simulink model "gear_motor"  (R2015a)
settings: Solver=ode45  StartTime=0.0  StopTime=180  FixedStep=0.01  RelTol=1e-3
libraries: dsparch4 x1
settings Model: Creator=keysie  LastModifiedBy=keysie
settings GRTTargetCC: RTWCAPISignals=on  RTWCAPIParams=on

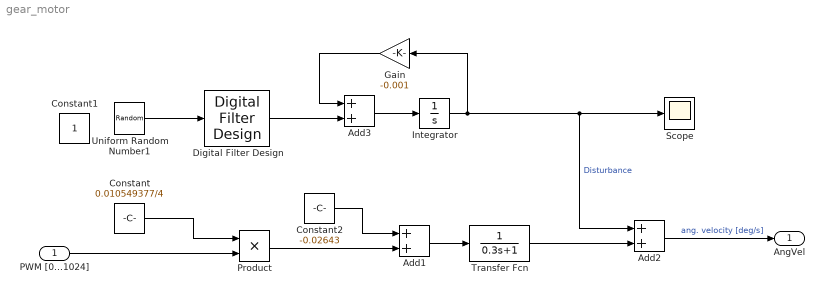
== system gear_motor ==
  PWM [0...1024] : Inport  Interpolate=off
  Add1 : Sum
  Add2 : Sum
  Add3 : Sum
  Constant : Constant  Value=0.010549377/4
  Constant2 : Constant  Value=-0.02643
  Digital Filter Design : dsparch4/Digital Filter Design  mwdsp_browser_bugfix_var=off
  Gain : Gain  Gain=-0.001
  Integrator : Integrator
  Product : Product
  Scope : Scope
  Transfer Fcn : TransferFcn  Denominator=[0.3 1]
  Uniform Random Number1 : UniformRandomNumber  Minimum=-0.02  Maximum=0.02  Seed=22324  SampleTime=0.1
  AngVel : Outport
  Constant1 : Constant  IOType=siggen
  wires:
  Constant/1 -> Product/1
  Constant2/1 -> Add1/1
  Product/1 -> Add1/2
  PWM [0...1024]/1 -> Product/2
  Add1/1 -> Transfer Fcn/1
  Integrator/1 -> Add2/1, Scope/1, Gain/1  "Disturbance"
  Add2/1 -> AngVel/1  "ang. velocity [deg/s]"
  Uniform Random Number1/1 -> Digital Filter Design/1
  Add3/1 -> Integrator/1
  Gain/1 -> Add3/1
  Transfer Fcn/1 -> Add2/2
  Digital Filter Design/1 -> Add3/2
